simulink model "MotorXploer"  (R2025a)
settings: Solver=FixedStepAuto  StartTime=0.0  StopTime=inf  FixedStep=0.001  RelTol=1e-3
undefined symbols (not defined in the file): Blocking, LF, Non
libraries: amg_usbconverter_n_connect_lib x3, dspxfrm3 x1, dspfdesign x1
settings Model: Creator=beamk  LastModifiedBy=fffif

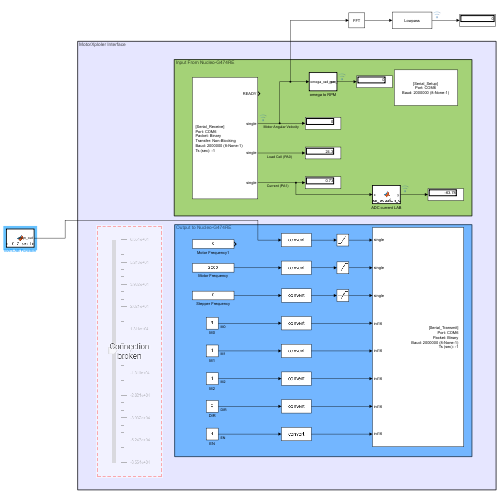
[thumbnail: Simulink's stored preview of the top-level diagram]
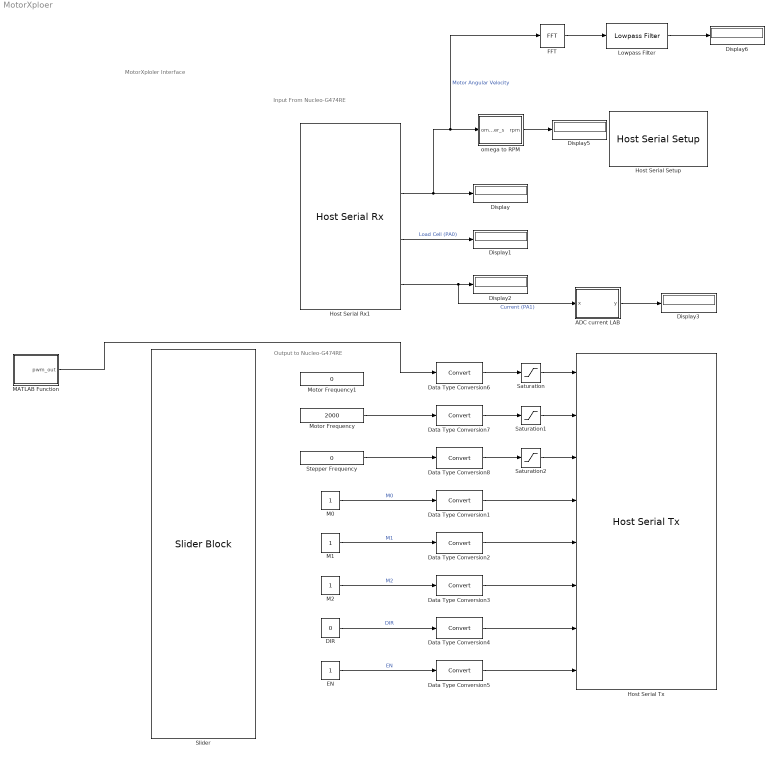
== system MotorXploer ==
  note: Output to Nucleo-G474RE
  note: Input From Nucleo-G474RE
  note: MotorXploler Interface
  ADC current LAB : MATLAB Function  TreatAsAtomicUnit=on
  DIR : Constant  Value=0
  Data Type Conversion{1..8} (8 alike) : DataTypeConversion  SaturateOnIntegerOverflow=off  RndMeth=Floor
  Display{,1..3,5..6} (6 alike) : Display
  EN : Constant
  FFT : dspxfrm3/FFT  FFTImplementation=Auto  CompMethod=Table lookup  TableOpt=NEW  TableOptActive=Speed  BitRevOrder=off  Normalize=off  InheritFFTLength=on  FFTLength=64  WrapInput=on  roundingMode=Ceiling  overflowMode=off  firstCoeffDataTypeStr=Inherit: Same word length as input  firstCoeffLastDataTypeStr=Inherit: Same word length as input  outputMin=[]  outputMax=[]
  Host Serial Rx1 : amg_usbconverter_n_connect_lib/Host Serial Rx  conf=rx  port=<auto>  baudrate=2000000  databits=8  parity=None  stopbit=1  flowcontrol=None  transfer=Non-Blocking  timeout=5  packetmode=Binary  enableinitialvalues=off  initialvalues=[]  binheader='25'  binterminator='4E'  porttype_double=0  porttype_single=3  porttype_int8=0  porttype_uint8=0  porttype_int16=0  porttype_uint16=0  porttype_int32=0  porttype_uint32=0  asciiformat='%f,%f,%d,%d'  rx_asciiterminator="LF (0x0A - \"\\n\")"  tx_asciiterminator="CRLF (0x0D 0x0A - \"\\r\\n\")"  sampletime=-1  enablecustomportlabel=off  cinputportlabel=0  coutputportlabel=A  portpinstr=0  blockid=HostSerialRx1  inputporttype=[]  inputportwidth=[]  inputportlabel={}  outputporttype=[3 1 1 1]  outputportwidth=[1 1 1 1]  outputportlabel={'READY','single','single','single'}  compat=0  optionstring=[]  autoport='COM6'
  Host Serial Setup : amg_usbconverter_n_connect_lib/Host Serial Setup  conf=setup  port=<auto>  baudrate=2000000  databits=8  parity=None  stopbit=1  flowcontrol=None  transfer=Blocking  timeout=2  packetmode=Binary  initialvalues=[]  binheader='7E 7E'  binterminator='03 03'  porttype_double=0  porttype_single=1  porttype_int8=0  porttype_uint8=0  porttype_int16=0  porttype_uint16=0  porttype_int32=0  porttype_uint32=2  asciiformat='%d %u %x'  rx_asciiterminator="CRLF (0x0D 0x0A - \"\\r\\n\")"  tx_asciiterminator="CRLF (0x0D 0x0A - \"\\r\\n\")"  sampletime=-1  enablecustomportlabel=off  cinputportlabel=0  coutputportlabel=A  portpinstr=0  blockid=HostSerialSetup  inputporttype=[]  inputportwidth=[]  inputportlabel={}  outputporttype=[]  outputportwidth=[]  outputportlabel={}  compat=0  optionstring=[]  autoport='COM6'
  Host Serial Tx : amg_usbconverter_n_connect_lib/Host Serial Tx  conf=tx  port=<auto>  baudrate=2000000  databits=8  parity=None  stopbit=1  flowcontrol=None  transfer=Blocking  timeout=2  packetmode=Binary  initialvalues=[]  binheader='25'  binterminator='4E'  porttype_double=0  porttype_single=3  porttype_int8=0  porttype_uint8=0  porttype_int16=5  porttype_uint16=0  porttype_int32=0  porttype_uint32=0  asciiformat='%d,%f'  rx_asciiterminator="CRLF (0x0D 0x0A - \"\\r\\n\")"  tx_asciiterminator="CRLF (0x0D 0x0A - \"\\r\\n\")"  sampletime=-1  enablecustomportlabel=off  cinputportlabel=0  coutputportlabel=A  portpinstr=0  blockid=HostSerialTx  inputporttype=[1 1 1 4 4 4 4 4]  inputportwidth=[1 1 1 1 1 1 1 1]  inputportlabel={'single','single','single','int16','int16','int16','int16','int16'}  outputporttype=[]  outputportwidth=[]  outputportlabel={}  compat=0  optionstring=[]  autoport='COM6'
      settings: SourceProductName=aMG USB Converter N
  Lowpass Filter : dspfdesign/Lowpass Filter  FilterType=FIR  DesignForMinimumOrder=on  FilterOrder=50  PassbandFrequency=0.3628  StopbandFrequency=0.5442  PassbandRipple=0.1  StopbandAttenuation=80  SampleRateMode=Use normalized frequency (0 to 1)  SampleRate=44100  SimulateUsing=Interpreted execution  roundingMode=Floor  coeffsDataTypeStr=fixdt(1,16)
  M0 : Constant
  M1 : Constant
  M2 : Constant
  MATLAB Function : MATLAB Function  TreatAsAtomicUnit=on
  Motor Frequency : Constant  Value=2000  OutDataTypeStr=single
  Motor Frequency1 : Constant  Value=0  VectorParams1D=off  OutDataTypeStr=single
  Saturation : Saturate  UpperLimit=65535  LowerLimit=-65535
  Saturation1 : Saturate  UpperLimit=20000  LowerLimit=0
  Saturation2 : Saturate  UpperLimit=inf  LowerLimit=0
  Slider : SliderBlock  ScaleMin=-65535  ScaleMax=65535
  Stepper Frequency : Constant  Value=0  OutDataTypeStr=single
  omega to RPM : MATLAB Function  TreatAsAtomicUnit=on
  wires:
  Host Serial Rx1/2 -> FFT/1, omega to RPM/1(omega_rad_per_s), Display/1  "Motor Angular Velocity"
  Host Serial Rx1/3 -> Display1/1  "Load Cell (PA0)"
  M0/1 -> Data Type Conversion1/1  "M0"
  EN/1 -> Data Type Conversion5/1  "EN"
  DIR/1 -> Data Type Conversion4/1  "DIR"
  M1/1 -> Data Type Conversion2/1  "M1"
  M2/1 -> Data Type Conversion3/1  "M2"
  Stepper Frequency/1 -> Data Type Conversion8/1
  Data Type Conversion1/1 -> Host Serial Tx/4
  Data Type Conversion2/1 -> Host Serial Tx/5
  Data Type Conversion3/1 -> Host Serial Tx/6
  Data Type Conversion4/1 -> Host Serial Tx/7
  Data Type Conversion5/1 -> Host Serial Tx/8
  Data Type Conversion6/1 -> Saturation/1
  Saturation/1 -> Host Serial Tx/1
  Data Type Conversion7/1 -> Saturation1/1
  Data Type Conversion8/1 -> Saturation2/1
  Saturation1/1 -> Host Serial Tx/2
  Saturation2/1 -> Host Serial Tx/3
  Host Serial Rx1/4 -> ADC current LAB/1(x), Display2/1  "Current (PA1)"
  ADC current LAB/1(y) -> Display3/1
  omega to RPM/1(rpm) -> Display5/1
  FFT/1 -> Lowpass Filter/1
  Lowpass Filter/1 -> Display6/1
  Motor Frequency/1 -> Data Type Conversion7/1
  MATLAB Function/1(pwm_out) -> Data Type Conversion6/1

== matlab function MotorXploer/ADC current LAB ==
  data: x input; y output
function y = linear_equation_calc(x)
%LINEAR_EQUATION_CALC คำนวณค่า y จากสมการเส้นตรง y = 0.0312*x - 63.8
%   
%   อินพุต:
%       x - ค่าตัวแปรอิสระ (สามารถเป็นค่าเดี่ยว, เวกเตอร์, หรืออาเรย์)
%
%   เอาท์พุต:
%       y - ค่าตัวแปรตามที่คำนวณได้ (จะมีขนาดเดียวกับ x)
%
%   ตัวอย่างการใช้งาน:
%       >> y_val = linear_equation_calc(100)
%       y_val = -60.6800
%
%       >> x_vec = [1000, 2000, 3000];
%       >> y_vec = linear_equation_calc(x_vec)
%       y_vec = [-32.6000    -1.4000   29.8000]

    % กำหนดค่าสัมประสิทธิ์ (Coefficient) และจุดตัดแกน y (Intercept)
    m = 0.0312; % ความชัน (Slope)
    b = -63.8;  % จุดตัดแกน y (Y-intercept)

    % คำนวณสมการเส้นตรง: y = m*x + b
    y = m .* x + b;
    
end

== matlab function MotorXploer/omega to RPM ==
  data: omega_rad_per_s input; rpm output
function rpm = angular_vel_to_rpm(omega_rad_per_s)
%ANGULAR_VEL_TO_RPM แปลง Angular Velocity (เรเดียนต่อวินาที) เป็น RPM
%
%   อินพุต:
%       omega_rad_per_s - ค่า Angular Velocity ในหน่วย rad/s (ค่าเดียว)
%
%   เอาท์พุต:
%       rpm - ค่า Rotations Per Minute (รอบต่อนาที) (ค่าเดียว)

    % ค่าคงที่ 60/(2*pi)
    conversion_factor = 60 / (2 * pi); 

    % คำนวณ RPM
    rpm = omega_rad_per_s * conversion_factor; % ใช้ * แทน .* เพราะรับค่าเดียว
    
end

== matlab function MotorXploer/MATLAB Function ==
  data: pwm_out output
function pwm_out = pwm_0_2_sec_timer()
%#codegen
% PWM_0_2_SEC_TIMER: สั่ง PWM MAX (65000) เป็นเวลา 0.2 วินาที แล้วหยุด (0)
%
%   เอาท์พุต:
%       pwm_out - ค่า PWM (65000 หรือ 0)
    
    %% --- 1. ตั้งค่าพารามิเตอร์ ---
    max_pwm_cnt = 65000;    % ค่า PWM สูงสุด
    
    % *** สมมติฐาน: อัตราการเรียกใช้ฟังก์ชัน (Sampling Frequency) ***
    % ต้องกำหนดอัตราการเรียกใช้เพื่อแปลง "นับ" เป็น "วินาที"
    sampling_freq = 1000;   % อัตราเรียกใช้ฟังก์ชัน (เช่น 1000 ครั้ง/วินาที หรือ 1 kHz)
    
    % คำนวณจำนวนรอบ (timer count) ที่ต้องนับเพื่อให้ครบ 0.2 วินาที
    run_duration_sec = 0.5; 
    max_count = run_duration_sec * sampling_freq; % 0.2 * 1000 = 200 รอบ
    
    %% --- 2. ตัวแปรจำค่า (Timer/x) ---
    % 'counter' ทำหน้าที่เป็นตัวนับเวลา (คล้ายกับ 'x' ในแนวคิดที่คุณเสนอ)
    persistent counter finished;
    
    if isempty(counter)
        % เริ่มต้น (ทำงานเพียงครั้งเดียว)
        counter = 0;
        finished = 0; % 0: กำลังทำงาน, 1: ทำงานเสร็จสิ้นแล้ว
    end
    
    %% --- 3. โลจิกควบคุมตาม Timer (x) ---
    % ถ้าตัวนับ (x/counter) ยังไม่ถึงขีดจำกัด (max_count/0.2 วิ)
    if finished == 1
        % A. จบแล้ว -> สั่งหยุด
        pwm_out = 0;
    elseif counter < max_count 
        % B. กำลังทำงาน 0.2 วินาที (Timer/x กำลังเดิน) -> สั่ง PWM สูงสุด
        pwm_out = max_pwm_cnt;
        % นับเวลา (เพิ่มค่า Timer/x)
        counter = counter + 1;
    else
        % C. ครบ 0.2 วินาทีแล้ว -> สั่งหยุดและตั้งค่าจบ
        pwm_out = 0;
        finished = 1;
    end
end
